simulink model "Dan1l"  (R2012b)
settings: Solver=ode45  StartTime=0.0  StopTime=10.0  RelTol=1e-3
undefined symbols (not defined in the file): Dan1
settings Model: Creator=Daniel  LastModifiedBy=Daniel

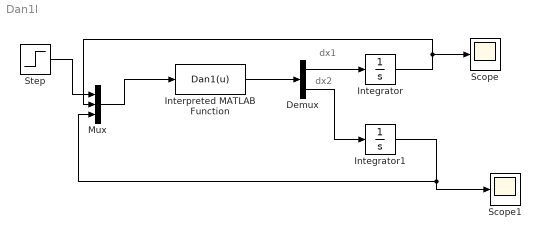
== system Dan1l ==
  note: dx2
  note: dx1
  Demux : Demux  Outputs=2
  Integrator : Integrator
  Integrator1 : Integrator
  Interpreted MATLAB Function : MATLABFcn  MATLABFcn=Dan1(u)  OutputDimensions=2
  Mux : Mux  Inputs=3
  Scope : Scope
  Scope1 : Scope
  Step : Step  After=18  SampleTime=0
  wires:
  Step/1 -> Mux/1
  Mux/1 -> Interpreted MATLAB Function/1
  Interpreted MATLAB Function/1 -> Demux/1
  Demux/2 -> Integrator1/1
  Demux/1 -> Integrator/1
  Integrator/1 -> Mux/2, Scope/1
  Integrator1/1 -> Mux/3, Scope1/1
